simulink model "Aearial_Inspection_UAV"  (R2021a)
settings: Solver=ode4  StartTime=0.0  StopTime=10.0  FixedStep=0.01  RelTol=1e-3
settings Model: SimulationMode=accelerator  Creator=mojta  LastModifiedBy=mojta

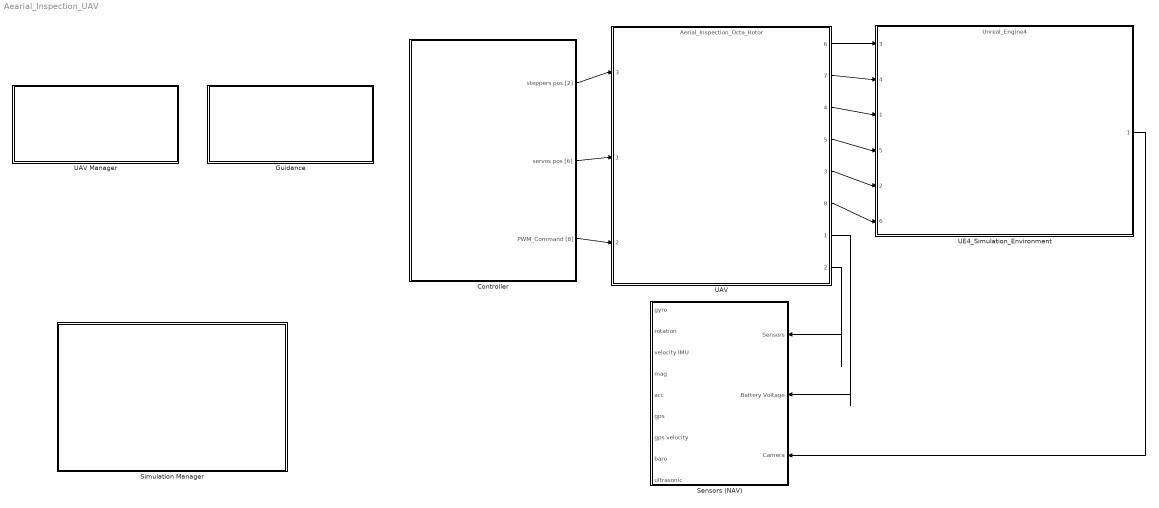
== system Aearial_Inspection_UAV ==
  Controller : Subsystem
      settings: PortSchema="{\"entries\":[{\"content\":{\"headerSize\":26,\"margin\":15,\"minimumSpacing\":25,\"sides\":[{\"content\":{\"connectorIds\":[]},\"type\":\"ConnectorPlacement.EquallySpacedRectSide\",\"uuid\":\"96273ddf-0f5d-40a8-85fb-f03d0280b449\"},{\"content\":{\"connectorIds\":[\"Out1\",\"Out2\",\"Out3\"],\"side\":\"RIGHT\"},\"type\":\"ConnectorPlacement.EquallySpacedRectSide\",\"uuid\":\"c880de00-51f9-4f30-9167-a4eda76e0d1f\"},{\"content\":{\"connectorIds\":[],\"side\":\"TOP\"},\"type\":\"ConnectorPlacement.EquallySpacedRectSide\",\"uuid\":\"fa2dd188-e601-4b4b-acde-a1f49a01b1f0\"},{\"content\":{\"connectorIds\":[],\"side\":\"BOTTOM\"},\"type\":\"ConnectorPlacement.EquallySpacedRectSide\",\"uuid\":\"d0783cfa-0613-4d0f-9a88-16370942cf45\"}]},\"type\":\"ConnectorPlacement.EquallySpacedConnector\",\"uuid\":\"457c6ef9-918c-42d9-985f-13d0159b3266\"}],\"packageUris\":[\"http://schema.mathworks.com/mf0/Connector/R2020b\"],\"version\":\"1.0\"}"
  Guidance : Subsystem
      settings: PortSchema="{\"entries\":[{\"content\":{\"headerSize\":26,\"margin\":15,\"minimumSpacing\":25,\"sides\":[{\"content\":{\"connectorIds\":[]},\"type\":\"ConnectorPlacement.EquallySpacedRectSide\",\"uuid\":\"96273ddf-0f5d-40a8-85fb-f03d0280b449\"},{\"content\":{\"connectorIds\":[],\"side\":\"RIGHT\"},\"type\":\"ConnectorPlacement.EquallySpacedRectSide\",\"uuid\":\"c880de00-51f9-4f30-9167-a4eda76e0d1f\"},{\"content\":{\"connectorIds\":[],\"side\":\"TOP\"},\"type\":\"ConnectorPlacement.EquallySpacedRectSide\",\"uuid\":\"fa2dd188-e601-4b4b-acde-a1f49a01b1f0\"}]},\"type\":\"ConnectorPlacement.EquallySpacedConnector\",\"uuid\":\"457c6ef9-918c-42d9-985f-13d0159b3266\"}],\"packageUris\":[\"http://schema.mathworks.com/mf0/Connector/R2020b\"],\"version\":\"1.0\"}"
  Sensors (NAV) : Subsystem
      settings: PortSchema="{\"entries\":[{\"content\":{\"headerSize\":26,\"margin\":15,\"minimumSpacing\":25,\"sides\":[{\"content\":{\"connectorIds\":[\"Out1\",\"Out2\",\"Out3\",\"Out4\",\"Out5\",\"Out6\",\"Out7\",\"Out8\",\"Out9\"]},\"type\":\"ConnectorPlacement.EquallySpacedRectSide\",\"uuid\":\"96273ddf-0f5d-40a8-85fb-f03d0280b449\"},{\"content\":{\"connectorIds\":[\"In2\",\"In1\",\"In3\"],\"side\":\"RIGHT\"},\"type\":\"ConnectorPlacement.EquallySpacedRectSide\",\"uuid\":\"c880de00-51f9-4f30-9167-a4eda76e0d1f\"},{\"content\":{\"connectorIds\":[],\"side\":\"TOP\"},\"type\":\"ConnectorPlacement.EquallySpacedRectSide\",\"uuid\":\"fa2dd188-e601-4b4b-acde-a1f49a01b1f0\"},{\"content\":{\"connectorIds\":[],\"side\":\"BOTTOM\"},\"type\":\"ConnectorPlacement.EquallySpacedRectSide\",\"uuid\":\"a7b7770f-59a4-4207-a1c0-248b9c805637\"}]},\"type\":\"ConnectorPlacement.EquallySpacedConnector\",\"uuid\":\"457c6ef9-918c-42d9-985f-13d0159b3266\"}],\"packageUris\":[\"http://schema.mathworks.com/mf0/Connector/R2020b\"],\"version\":\"1.0\"}"
  Simulation Manager : Subsystem
      settings: PortSchema="{\"entries\":[{\"content\":{\"headerSize\":26,\"margin\":15,\"minimumSpacing\":25,\"sides\":[{\"content\":{\"connectorIds\":[]},\"type\":\"ConnectorPlacement.EquallySpacedRectSide\",\"uuid\":\"96273ddf-0f5d-40a8-85fb-f03d0280b449\"},{\"content\":{\"connectorIds\":[],\"side\":\"RIGHT\"},\"type\":\"ConnectorPlacement.EquallySpacedRectSide\",\"uuid\":\"c880de00-51f9-4f30-9167-a4eda76e0d1f\"},{\"content\":{\"connectorIds\":[],\"side\":\"TOP\"},\"type\":\"ConnectorPlacement.EquallySpacedRectSide\",\"uuid\":\"fa2dd188-e601-4b4b-acde-a1f49a01b1f0\"}]},\"type\":\"ConnectorPlacement.EquallySpacedConnector\",\"uuid\":\"457c6ef9-918c-42d9-985f-13d0159b3266\"}],\"packageUris\":[\"http://schema.mathworks.com/mf0/Connector/R2020b\"],\"version\":\"1.0\"}"
  UAV : ModelReference  ModelNameDialog=Aerial_Inspection_Octa_Rotor.slx  SimulationMode=Normal  ModelReferenceVersion=1.35
      settings: PortSchema="{\"entries\":[{\"content\":{\"headerSize\":38,\"margin\":15,\"minimumSpacing\":25,\"sides\":[{\"content\":{\"connectorIds\":[\"In3\",\"In1\",\"In2\"]},\"type\":\"ConnectorPlacement.EquallySpacedRectSide\",\"uuid\":\"1389eede-0687-4233-acf3-c4e0e627e4f1\"},{\"content\":{\"connectorIds\":[\"Out6\",\"Out7\",\"Out4\",\"Out5\",\"Out3\",\"Out8\",\"Out1\",\"Out2\"],\"side\":\"RIGHT\"},\"type\":\"ConnectorPlacement.EquallySpacedRectSide\",\"uuid\":\"39c19b5f-b581-42cb-919d-1385d52af384\"},{\"content\":{\"connectorIds\":[],\"side\":\"TOP\"},\"type\":\"ConnectorPlacement.EquallySpacedRectSide\",\"uuid\":\"bc9bd074-aed9-46e3-b245-de97ec288fd2\"}]},\"type\":\"ConnectorPlacement.EquallySpacedConnector\",\"uuid\":\"487467df-dab5-429d-9ff2-066ab2a0fb04\"}],\"packageUris\":[\"http://schema.mathworks.com/mf0/Connector/R2020b\"],\"version\":\"1.0\"}"
  UAV Manager : Subsystem
      settings: PortSchema="{\"entries\":[{\"content\":{\"headerSize\":26,\"margin\":15,\"minimumSpacing\":25,\"sides\":[{\"content\":{\"connectorIds\":[]},\"type\":\"ConnectorPlacement.EquallySpacedRectSide\",\"uuid\":\"96273ddf-0f5d-40a8-85fb-f03d0280b449\"},{\"content\":{\"connectorIds\":[],\"side\":\"RIGHT\"},\"type\":\"ConnectorPlacement.EquallySpacedRectSide\",\"uuid\":\"c880de00-51f9-4f30-9167-a4eda76e0d1f\"},{\"content\":{\"connectorIds\":[],\"side\":\"TOP\"},\"type\":\"ConnectorPlacement.EquallySpacedRectSide\",\"uuid\":\"fa2dd188-e601-4b4b-acde-a1f49a01b1f0\"}]},\"type\":\"ConnectorPlacement.EquallySpacedConnector\",\"uuid\":\"457c6ef9-918c-42d9-985f-13d0159b3266\"}],\"packageUris\":[\"http://schema.mathworks.com/mf0/Connector/R2020b\"],\"version\":\"1.0\"}"
  UE4_Simulation_Environment : ModelReference  ModelNameDialog=Unreal_Engine4.slx  SimulationMode=Normal  ModelReferenceVersion=1.16
      settings: PortSchema="{\"entries\":[{\"content\":{\"headerSize\":38,\"margin\":15,\"minimumSpacing\":25,\"sides\":[{\"content\":{\"connectorIds\":[\"In3\",\"In4\",\"In1\",\"In5\",\"In2\",\"In6\"]},\"type\":\"ConnectorPlacement.EquallySpacedRectSide\",\"uuid\":\"1389eede-0687-4233-acf3-c4e0e627e4f1\"},{\"content\":{\"connectorIds\":[\"Out1\"],\"side\":\"RIGHT\"},\"type\":\"ConnectorPlacement.EquallySpacedRectSide\",\"uuid\":\"39c19b5f-b581-42cb-919d-1385d52af384\"},{\"content\":{\"connectorIds\":[],\"side\":\"TOP\"},\"type\":\"ConnectorPlacement.EquallySpacedRectSide\",\"uuid\":\"bc9bd074-aed9-46e3-b245-de97ec288fd2\"},{\"content\":{\"connectorIds\":[],\"side\":\"BOTTOM\"},\"type\":\"ConnectorPlacement.EquallySpacedRectSide\",\"uuid\":\"8d14421a-634b-4724-974a-7c39bddd1c49\"}]},\"type\":\"ConnectorPlacement.EquallySpacedConnector\",\"uuid\":\"487467df-dab5-429d-9ff2-066ab2a0fb04\"}],\"packageUris\":[\"http://schema.mathworks.com/mf0/Connector/R2020b\"],\"version\":\"1.0\"}"
  wires:
  UAV/2 -> Sensors (NAV)/2(Sensors)
  Controller/1(steppers pos [2]) -> UAV/3
  Controller/2(servos pos [6]) -> UAV/1
  Controller/3(PWM_Command [8]) -> UAV/2
  UAV/1 -> Sensors (NAV)/1(Battery Voltage)
  UAV/6 -> UE4_Simulation_Environment/3
  UAV/7 -> UE4_Simulation_Environment/4
  UAV/4 -> UE4_Simulation_Environment/1
  UAV/5 -> UE4_Simulation_Environment/5
  UAV/3 -> UE4_Simulation_Environment/2
  UE4_Simulation_Environment/1 -> Sensors (NAV)/3(Camera)
  UAV/8 -> UE4_Simulation_Environment/6

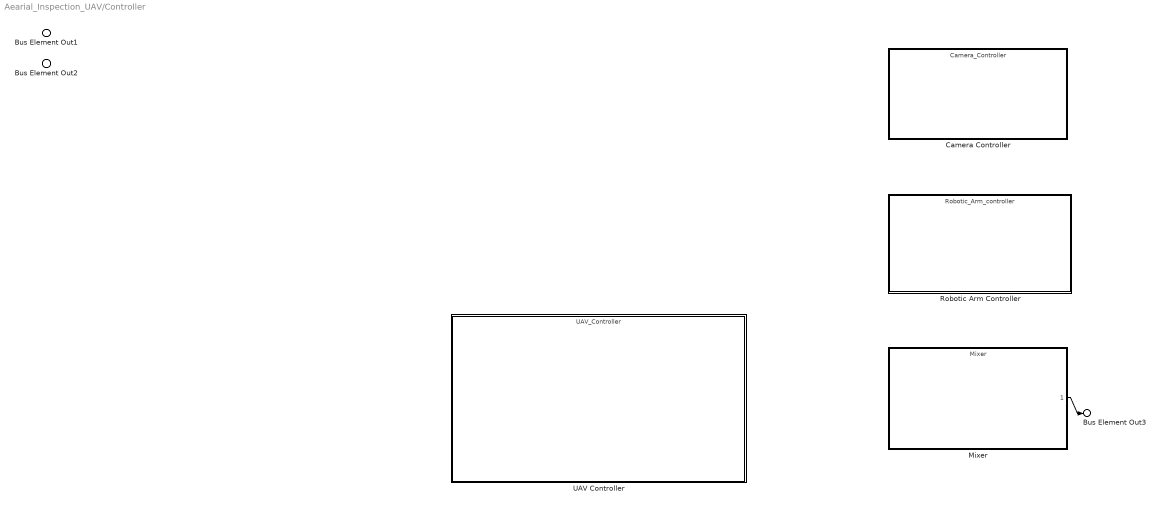
== system Aearial_Inspection_UAV/Controller ==
  Camera Controller : ModelReference  ModelNameDialog=Camera_Controller.slx  SimulationMode=Normal  ModelReferenceVersion=1.0
      settings: PortSchema="{\"entries\":[{\"content\":{\"headerSize\":38,\"margin\":15,\"minimumSpacing\":25,\"sides\":[{\"content\":{\"connectorIds\":[]},\"type\":\"ConnectorPlacement.EquallySpacedRectSide\",\"uuid\":\"1389eede-0687-4233-acf3-c4e0e627e4f1\"},{\"content\":{\"connectorIds\":[],\"side\":\"RIGHT\"},\"type\":\"ConnectorPlacement.EquallySpacedRectSide\",\"uuid\":\"39c19b5f-b581-42cb-919d-1385d52af384\"},{\"content\":{\"connectorIds\":[],\"side\":\"TOP\"},\"type\":\"ConnectorPlacement.EquallySpacedRectSide\",\"uuid\":\"bc9bd074-aed9-46e3-b245-de97ec288fd2\"}]},\"type\":\"ConnectorPlacement.EquallySpacedConnector\",\"uuid\":\"487467df-dab5-429d-9ff2-066ab2a0fb04\"}],\"packageUris\":[\"http://schema.mathworks.com/mf0/Connector/R2020b\"],\"version\":\"1.0\"}"
  Mixer : ModelReference  ModelNameDialog=Mixer.slx  SimulationMode=Normal  ModelReferenceVersion=1.1
      settings: PortSchema="{\"entries\":[{\"content\":{\"headerSize\":38,\"margin\":15,\"minimumSpacing\":25,\"sides\":[{\"content\":{\"connectorIds\":[]},\"type\":\"ConnectorPlacement.EquallySpacedRectSide\",\"uuid\":\"1389eede-0687-4233-acf3-c4e0e627e4f1\"},{\"content\":{\"connectorIds\":[\"Out1\"],\"side\":\"RIGHT\"},\"type\":\"ConnectorPlacement.EquallySpacedRectSide\",\"uuid\":\"39c19b5f-b581-42cb-919d-1385d52af384\"},{\"content\":{\"connectorIds\":[],\"side\":\"TOP\"},\"type\":\"ConnectorPlacement.EquallySpacedRectSide\",\"uuid\":\"bc9bd074-aed9-46e3-b245-de97ec288fd2\"}]},\"type\":\"ConnectorPlacement.EquallySpacedConnector\",\"uuid\":\"487467df-dab5-429d-9ff2-066ab2a0fb04\"}],\"packageUris\":[\"http://schema.mathworks.com/mf0/Connector/R2020b\"],\"version\":\"1.0\"}"
  Robotic Arm Controller : ModelReference  ModelNameDialog=Robotic_Arm_controller.slx  SimulationMode=Normal  ModelReferenceVersion=1.0
      settings: PortSchema="{\"entries\":[{\"content\":{\"headerSize\":38,\"margin\":15,\"minimumSpacing\":25,\"sides\":[{\"content\":{\"connectorIds\":[]},\"type\":\"ConnectorPlacement.EquallySpacedRectSide\",\"uuid\":\"1389eede-0687-4233-acf3-c4e0e627e4f1\"},{\"content\":{\"connectorIds\":[],\"side\":\"RIGHT\"},\"type\":\"ConnectorPlacement.EquallySpacedRectSide\",\"uuid\":\"39c19b5f-b581-42cb-919d-1385d52af384\"},{\"content\":{\"connectorIds\":[],\"side\":\"TOP\"},\"type\":\"ConnectorPlacement.EquallySpacedRectSide\",\"uuid\":\"bc9bd074-aed9-46e3-b245-de97ec288fd2\"}]},\"type\":\"ConnectorPlacement.EquallySpacedConnector\",\"uuid\":\"487467df-dab5-429d-9ff2-066ab2a0fb04\"}],\"packageUris\":[\"http://schema.mathworks.com/mf0/Connector/R2020b\"],\"version\":\"1.0\"}"
  UAV Controller : ModelReference  ModelNameDialog=UAV_Controller.slx  SimulationMode=Normal  ModelReferenceVersion=1.0
      settings: PortSchema="{\"entries\":[{\"content\":{\"headerSize\":38,\"margin\":15,\"minimumSpacing\":25,\"sides\":[{\"content\":{\"connectorIds\":[]},\"type\":\"ConnectorPlacement.EquallySpacedRectSide\",\"uuid\":\"1389eede-0687-4233-acf3-c4e0e627e4f1\"},{\"content\":{\"connectorIds\":[],\"side\":\"RIGHT\"},\"type\":\"ConnectorPlacement.EquallySpacedRectSide\",\"uuid\":\"39c19b5f-b581-42cb-919d-1385d52af384\"},{\"content\":{\"connectorIds\":[],\"side\":\"TOP\"},\"type\":\"ConnectorPlacement.EquallySpacedRectSide\",\"uuid\":\"bc9bd074-aed9-46e3-b245-de97ec288fd2\"}]},\"type\":\"ConnectorPlacement.EquallySpacedConnector\",\"uuid\":\"487467df-dab5-429d-9ff2-066ab2a0fb04\"}],\"packageUris\":[\"http://schema.mathworks.com/mf0/Connector/R2020b\"],\"version\":\"1.0\"}"
  Bus Element Out1 : Outport  PortName=steppers pos [2]
  Bus Element Out2 : Outport  Port=2  PortName=servos pos [6]
  Bus Element Out3 : Outport  Port=3  PortName=PWM_Command [8]
  wires:
  Mixer/1 -> Bus Element Out3/1

== system Aearial_Inspection_UAV/Guidance ==

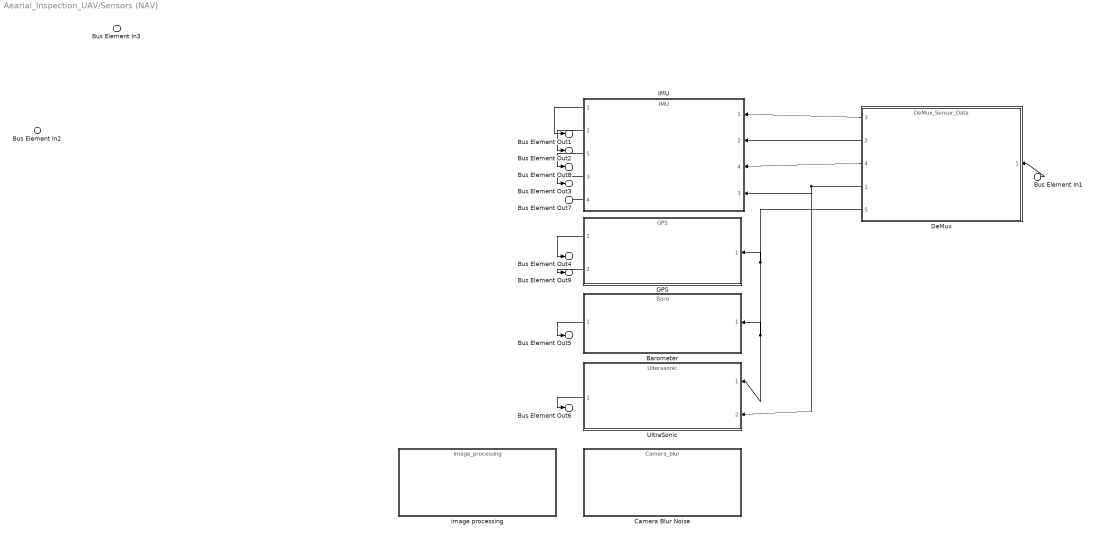
== system Aearial_Inspection_UAV/Sensors (NAV) ==
  Bus Element In3 : Inport  PortName=Battery Voltage
  Bus Element In1 : Inport  Port=2  PortName=Sensors
  Bus Element In2 : Inport  Port=3  PortName=Camera
  Barometer : ModelReference  ModelNameDialog=Baro.slx  SimulationMode=Normal  ModelReferenceVersion=1.5
      settings: PortSchema="{\"entries\":[{\"content\":{\"headerSize\":38,\"margin\":15,\"minimumSpacing\":25,\"sides\":[{\"content\":{\"connectorIds\":[\"Out1\"]},\"type\":\"ConnectorPlacement.EquallySpacedRectSide\",\"uuid\":\"1389eede-0687-4233-acf3-c4e0e627e4f1\"},{\"content\":{\"connectorIds\":[\"In1\"],\"side\":\"RIGHT\"},\"type\":\"ConnectorPlacement.EquallySpacedRectSide\",\"uuid\":\"39c19b5f-b581-42cb-919d-1385d52af384\"},{\"content\":{\"connectorIds\":[],\"side\":\"TOP\"},\"type\":\"ConnectorPlacement.EquallySpacedRectSide\",\"uuid\":\"bc9bd074-aed9-46e3-b245-de97ec288fd2\"},{\"content\":{\"connectorIds\":[],\"side\":\"BOTTOM\"},\"type\":\"ConnectorPlacement.EquallySpacedRectSide\",\"uuid\":\"66df8d0b-587f-46b3-96c4-fa9d7ec5f44d\"}]},\"type\":\"ConnectorPlacement.EquallySpacedConnector\",\"uuid\":\"487467df-dab5-429d-9ff2-066ab2a0fb04\"}],\"packageUris\":[\"http://schema.mathworks.com/mf0/Connector/R2020b\"],\"version\":\"1.0\"}"
  Camera Blur Noise : ModelReference  ModelNameDialog=Camera_blur.slx  SimulationMode=Normal  ModelReferenceVersion=1.0
      settings: PortSchema="{\"entries\":[{\"content\":{\"headerSize\":38,\"margin\":15,\"minimumSpacing\":25,\"sides\":[{\"content\":{\"connectorIds\":[]},\"type\":\"ConnectorPlacement.EquallySpacedRectSide\",\"uuid\":\"1389eede-0687-4233-acf3-c4e0e627e4f1\"},{\"content\":{\"connectorIds\":[],\"side\":\"RIGHT\"},\"type\":\"ConnectorPlacement.EquallySpacedRectSide\",\"uuid\":\"39c19b5f-b581-42cb-919d-1385d52af384\"},{\"content\":{\"connectorIds\":[],\"side\":\"TOP\"},\"type\":\"ConnectorPlacement.EquallySpacedRectSide\",\"uuid\":\"bc9bd074-aed9-46e3-b245-de97ec288fd2\"},{\"content\":{\"connectorIds\":[],\"side\":\"BOTTOM\"},\"type\":\"ConnectorPlacement.EquallySpacedRectSide\",\"uuid\":\"bc26ae2f-6e68-4422-98ec-21b46d7a754b\"}]},\"type\":\"ConnectorPlacement.EquallySpacedConnector\",\"uuid\":\"487467df-dab5-429d-9ff2-066ab2a0fb04\"}],\"packageUris\":[\"http://schema.mathworks.com/mf0/Connector/R2020b\"],\"version\":\"1.0\"}"
  DeMux : ModelReference  ModelNameDialog=DeMux_Sensor_Data.slx  SimulationMode=Normal  ModelReferenceVersion=1.6
      settings: PortSchema="{\"entries\":[{\"content\":{\"headerSize\":38,\"margin\":15,\"minimumSpacing\":25,\"sides\":[{\"content\":{\"connectorIds\":[\"Out3\",\"Out2\",\"Out4\",\"Out1\",\"Out5\"]},\"type\":\"ConnectorPlacement.EquallySpacedRectSide\",\"uuid\":\"1389eede-0687-4233-acf3-c4e0e627e4f1\"},{\"content\":{\"connectorIds\":[\"In1\"],\"side\":\"RIGHT\"},\"type\":\"ConnectorPlacement.EquallySpacedRectSide\",\"uuid\":\"39c19b5f-b581-42cb-919d-1385d52af384\"},{\"content\":{\"connectorIds\":[],\"side\":\"TOP\"},\"type\":\"ConnectorPlacement.EquallySpacedRectSide\",\"uuid\":\"bc9bd074-aed9-46e3-b245-de97ec288fd2\"},{\"content\":{\"connectorIds\":[],\"side\":\"BOTTOM\"},\"type\":\"ConnectorPlacement.EquallySpacedRectSide\",\"uuid\":\"ae4f97c5-3a70-4f2e-8d12-7a37e2efe99a\"}]},\"type\":\"ConnectorPlacement.EquallySpacedConnector\",\"uuid\":\"487467df-dab5-429d-9ff2-066ab2a0fb04\"}],\"packageUris\":[\"http://schema.mathworks.com/mf0/Connector/R2020b\"],\"version\":\"1.0\"}"
  GPS : ModelReference  ModelNameDialog=GPS.slx  SimulationMode=Normal  ModelReferenceVersion=1.6
      settings: PortSchema="{\"entries\":[{\"content\":{\"headerSize\":38,\"margin\":15,\"minimumSpacing\":25,\"sides\":[{\"content\":{\"connectorIds\":[\"Out1\",\"Out2\"]},\"type\":\"ConnectorPlacement.EquallySpacedRectSide\",\"uuid\":\"1389eede-0687-4233-acf3-c4e0e627e4f1\"},{\"content\":{\"connectorIds\":[\"In1\"],\"side\":\"RIGHT\"},\"type\":\"ConnectorPlacement.EquallySpacedRectSide\",\"uuid\":\"39c19b5f-b581-42cb-919d-1385d52af384\"},{\"content\":{\"connectorIds\":[],\"side\":\"TOP\"},\"type\":\"ConnectorPlacement.EquallySpacedRectSide\",\"uuid\":\"bc9bd074-aed9-46e3-b245-de97ec288fd2\"},{\"content\":{\"connectorIds\":[],\"side\":\"BOTTOM\"},\"type\":\"ConnectorPlacement.EquallySpacedRectSide\",\"uuid\":\"b5ee566b-4511-42aa-a01d-703eb3d04952\"}]},\"type\":\"ConnectorPlacement.EquallySpacedConnector\",\"uuid\":\"487467df-dab5-429d-9ff2-066ab2a0fb04\"}],\"packageUris\":[\"http://schema.mathworks.com/mf0/Connector/R2020b\"],\"version\":\"1.0\"}"
  IMU : ModelReference  ModelNameDialog=IMU.slx  SimulationMode=Normal  ModelReferenceVersion=1.12
      settings: PortSchema="{\"entries\":[{\"content\":{\"headerSize\":38,\"margin\":15,\"minimumSpacing\":25,\"sides\":[{\"content\":{\"connectorIds\":[\"Out1\",\"Out2\",\"Out5\",\"Out3\",\"Out4\"]},\"type\":\"ConnectorPlacement.EquallySpacedRectSide\",\"uuid\":\"1389eede-0687-4233-acf3-c4e0e627e4f1\"},{\"content\":{\"connectorIds\":[\"In1\",\"In2\",\"In4\",\"In3\"],\"side\":\"RIGHT\"},\"type\":\"ConnectorPlacement.EquallySpacedRectSide\",\"uuid\":\"39c19b5f-b581-42cb-919d-1385d52af384\"},{\"content\":{\"connectorIds\":[],\"side\":\"TOP\"},\"type\":\"ConnectorPlacement.EquallySpacedRectSide\",\"uuid\":\"bc9bd074-aed9-46e3-b245-de97ec288fd2\"},{\"content\":{\"connectorIds\":[],\"side\":\"BOTTOM\"},\"type\":\"ConnectorPlacement.EquallySpacedRectSide\",\"uuid\":\"6d8703c9-9862-4a6a-9947-d765cc5a6fa1\"}]},\"type\":\"ConnectorPlacement.EquallySpacedConnector\",\"uuid\":\"487467df-dab5-429d-9ff2-066ab2a0fb04\"}],\"packageUris\":[\"http://schema.mathworks.com/mf0/Connector/R2020b\"],\"version\":\"1.0\"}"
  UltraSonic : ModelReference  ModelNameDialog=Ulterasonic.slx  SimulationMode=Normal  ModelReferenceVersion=1.47
      settings: PortSchema="{\"entries\":[{\"content\":{\"headerSize\":38,\"margin\":15,\"minimumSpacing\":25,\"sides\":[{\"content\":{\"connectorIds\":[\"Out1\"]},\"type\":\"ConnectorPlacement.EquallySpacedRectSide\",\"uuid\":\"1389eede-0687-4233-acf3-c4e0e627e4f1\"},{\"content\":{\"connectorIds\":[\"In1\",\"In2\"],\"side\":\"RIGHT\"},\"type\":\"ConnectorPlacement.EquallySpacedRectSide\",\"uuid\":\"39c19b5f-b581-42cb-919d-1385d52af384\"},{\"content\":{\"connectorIds\":[],\"side\":\"TOP\"},\"type\":\"ConnectorPlacement.EquallySpacedRectSide\",\"uuid\":\"bc9bd074-aed9-46e3-b245-de97ec288fd2\"},{\"content\":{\"connectorIds\":[],\"side\":\"BOTTOM\"},\"type\":\"ConnectorPlacement.EquallySpacedRectSide\",\"uuid\":\"38340f11-5211-4009-810b-363b7ea9b66f\"}]},\"type\":\"ConnectorPlacement.EquallySpacedConnector\",\"uuid\":\"487467df-dab5-429d-9ff2-066ab2a0fb04\"}],\"packageUris\":[\"http://schema.mathworks.com/mf0/Connector/R2020b\"],\"version\":\"1.0\"}"
  image processing : ModelReference  ModelNameDialog=image_processing.slx  SimulationMode=Normal  ModelReferenceVersion=1.0
      settings: PortSchema="{\"entries\":[{\"content\":{\"headerSize\":38,\"margin\":15,\"minimumSpacing\":25,\"sides\":[{\"content\":{\"connectorIds\":[]},\"type\":\"ConnectorPlacement.EquallySpacedRectSide\",\"uuid\":\"1389eede-0687-4233-acf3-c4e0e627e4f1\"},{\"content\":{\"connectorIds\":[],\"side\":\"RIGHT\"},\"type\":\"ConnectorPlacement.EquallySpacedRectSide\",\"uuid\":\"39c19b5f-b581-42cb-919d-1385d52af384\"},{\"content\":{\"connectorIds\":[],\"side\":\"TOP\"},\"type\":\"ConnectorPlacement.EquallySpacedRectSide\",\"uuid\":\"bc9bd074-aed9-46e3-b245-de97ec288fd2\"},{\"content\":{\"connectorIds\":[],\"side\":\"BOTTOM\"},\"type\":\"ConnectorPlacement.EquallySpacedRectSide\",\"uuid\":\"7e078513-cf78-4d1a-88c2-56bb86b4860e\"}]},\"type\":\"ConnectorPlacement.EquallySpacedConnector\",\"uuid\":\"487467df-dab5-429d-9ff2-066ab2a0fb04\"}],\"packageUris\":[\"http://schema.mathworks.com/mf0/Connector/R2020b\"],\"version\":\"1.0\"}"
  Bus Element Out1 : Outport  PortName=gyro
  Bus Element Out7 : Outport  Port=2  PortName=rotation
  Bus Element Out8 : Outport  Port=3  PortName=velocity IMU
  Bus Element Out3 : Outport  Port=4  PortName=mag
  Bus Element Out2 : Outport  Port=5  PortName=acc
  Bus Element Out4 : Outport  Port=6  PortName=gps
  Bus Element Out9 : Outport  Port=7  PortName=gps velocity
  Bus Element Out5 : Outport  Port=8  PortName=baro
  Bus Element Out6 : Outport  Port=9  PortName=ultrasonic
  wires:
  DeMux/3 -> IMU/1
  DeMux/2 -> IMU/2
  Bus Element In1/1 -> DeMux/1
  DeMux/5 -> UltraSonic/1, Barometer/1, GPS/1
  IMU/2 -> Bus Element Out2/1
  IMU/3 -> Bus Element Out3/1
  GPS/1 -> Bus Element Out4/1
  Barometer/1 -> Bus Element Out5/1
  UltraSonic/1 -> Bus Element Out6/1
  IMU/1 -> Bus Element Out1/1
  DeMux/1 -> UltraSonic/2, IMU/3
  IMU/4 -> Bus Element Out7/1
  DeMux/4 -> IMU/4
  IMU/5 -> Bus Element Out8/1
  GPS/2 -> Bus Element Out9/1

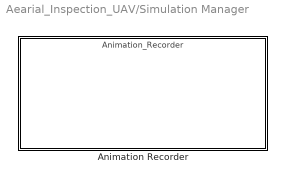
== system Aearial_Inspection_UAV/Simulation Manager ==
  Animation Recorder : ModelReference  ModelNameDialog=Animation_Recorder.slx  SimulationMode=Normal  ModelReferenceVersion=1.2
      settings: PortSchema="{\"entries\":[{\"content\":{\"headerSize\":38,\"margin\":15,\"minimumSpacing\":25,\"sides\":[{\"content\":{\"connectorIds\":[]},\"type\":\"ConnectorPlacement.EquallySpacedRectSide\",\"uuid\":\"901e70cd-68e1-4e4e-b2bb-a76a839cfc12\"},{\"content\":{\"connectorIds\":[],\"side\":\"RIGHT\"},\"type\":\"ConnectorPlacement.EquallySpacedRectSide\",\"uuid\":\"fa2f2a46-70a9-4c8a-971b-0d22cace0a49\"},{\"content\":{\"connectorIds\":[],\"side\":\"TOP\"},\"type\":\"ConnectorPlacement.EquallySpacedRectSide\",\"uuid\":\"5ce954cb-c23a-4703-a9b6-32272cc88152\"}]},\"type\":\"ConnectorPlacement.EquallySpacedConnector\",\"uuid\":\"25f92397-ee4d-47a9-8cb1-d8870df7685d\"}],\"packageUris\":[\"http://schema.mathworks.com/mf0/Connector/R2020b\"],\"version\":\"1.0\"}"

== system Aearial_Inspection_UAV/UAV Manager ==
